simulink model "ssm"  (R2017b)
settings: Solver=FixedStepDiscrete  StartTime=0.0  StopTime=20  FixedStep=T_s_power  MaxStep=1e-4  RelTol=1e-3
values from neighbouring files (symbols this model uses):
  F_b = 50.0    (= 50)    [ssm_ini.m]
  L_1 = 10e-3    (= 0.01)    [ssm_ini.m]
  L_2 = 1e-3    (= 0.001)    [ssm_ini.m]
  Omega_b = 2*pi*50    (= 314.159265359)    [ssm_ini.m]
  params_abc = [S_b,U_b,Omega_b,K,K_d]    [ssm_ini.m]
  params_pll = [K_p,Omega_b]    [ssm_ini.m]
  params_pu = [S_b,U_b,Omega_b,R_pu,X_pu,H,D]    [ssm_ini.m]
  R_1 = 1.0    (= 1)    [ssm_ini.m]
  R_2 = 1.0    (= 1)    [ssm_ini.m]
  S_b = 20e3    (= 20000)    [ssm_ini.m]
  T_s_control = 100e-6    (= 0.0001)    [ssm_ini.m]
  T_s_power = 100e-6    (= 0.0001)    [ssm_ini.m]
undefined symbols (not defined in the file or in its folder): DiscIntNeverNeededParam
libraries: powerlib x18, powerlib_meascontrol x6
settings Model: Creator=jmmauricio  LastModifiedBy=jmmau
settings CodeAppCC: StateflowObjectComments=on
settings SimscapeCC: SimscapeNormalizeSystem=off

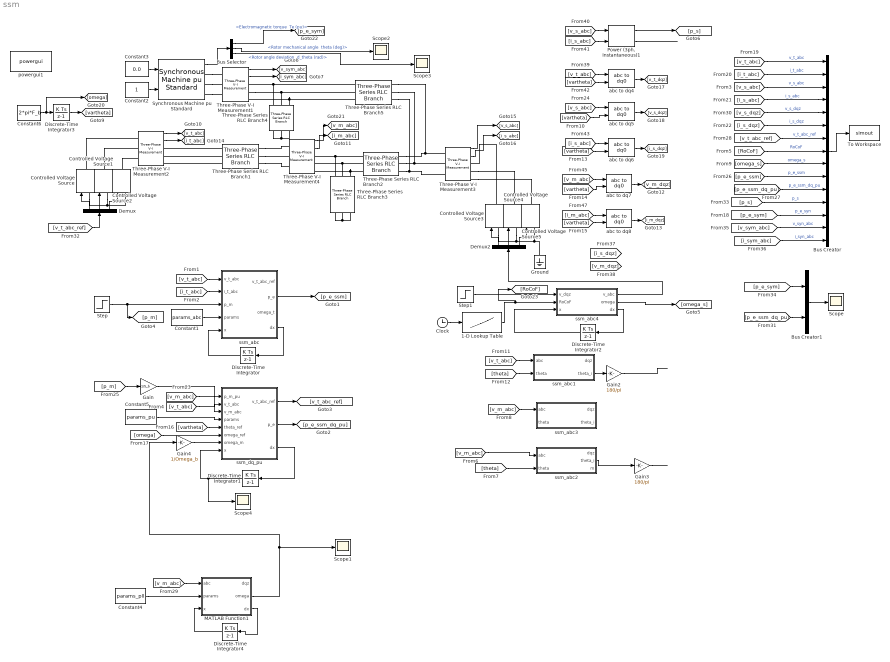
== system ssm ==
  1-D Lookup Table : Lookup_n-D  NumberOfTableDimensions=1  BreakpointsForDimension1=[0,1,1.01,6.0,6.01,15]+5  Table=[0,0,-1,-1,0,0]  InternalRulePriority=Speed  RndMeth=Simplest  InputSameDT=on
  Bus Creator : BusCreator  Inputs=15
  Bus Creator1 : BusCreator  Inputs=2
  Bus Selector : BusSelector  OutputSignals="Mechanical.Electromagnetic torque  Te (pu),Mechanical.Rotor mechanical angle  theta (deg),Mechanical.Rotor angle deviation  d_theta (rad)"
  Clock : Clock
  Constant1 : Constant  Value=params_abc
  Constant2 : Constant
  Constant3 : Constant  Value=0.0
  Constant4 : Constant  Value=params_pll
  Constant5 : Constant  Value=params_pu
  Constant6 : Constant  Value=2*pi*F_b
  Controlled Voltage Source{,1..5} (6 alike) : powerlib/Electrical Sources/Controlled Voltage Source  Initialize=on  Source_Type=AC  Amplitude=0  Phase=0  Frequency=0  Measurements=None
  Demux : Demux  Outputs=3
  Demux2 : Demux  Outputs=3
  Discrete-Time Integrator : DiscreteIntegrator  InitialCondition=[0,Omega_b]  InitialConditionSetting=State (most efficient)  SampleTime=T_s_power  ICPrevOutput=DiscIntNeverNeededParam  ICPrevScaledInput=DiscIntNeverNeededParam
  Discrete-Time Integrator1 : DiscreteIntegrator  InitialCondition=[0,1,0]  InitialConditionSetting=State (most efficient)  SampleTime=T_s_control  ICPrevOutput=DiscIntNeverNeededParam  ICPrevScaledInput=DiscIntNeverNeededParam
  Discrete-Time Integrator2 : DiscreteIntegrator  InitialCondition=[0,Omega_b]  InitialConditionSetting=State (most efficient)  SampleTime=T_s_power  ICPrevOutput=DiscIntNeverNeededParam  ICPrevScaledInput=DiscIntNeverNeededParam
  Discrete-Time Integrator3 : DiscreteIntegrator  InitialConditionSetting=State (most efficient)  SampleTime=T_s_power  ICPrevOutput=DiscIntNeverNeededParam  ICPrevScaledInput=DiscIntNeverNeededParam
  Discrete-Time Integrator4 : DiscreteIntegrator  InitialConditionSetting=State (most efficient)  SampleTime=T_s_power  ICPrevOutput=DiscIntNeverNeededParam  ICPrevScaledInput=DiscIntNeverNeededParam
  Gain : Gain  Gain=1/S_b
  Gain2 : Gain  Gain=180/pi
  Gain3 : Gain  Gain=180/pi
  Gain4 : Gain  Gain=1/Omega_b
  Ground : powerlib/Elements/Ground  LConnTagsString=a
  MATLAB Function1 : MATLAB Function  TreatAsAtomicUnit=on
  "Power (3ph, Instantaneous)1" : powerlib_meascontrol/Measurements/Power (3ph, Instantaneous)
      settings: SourceProductName=Simscape Power Systems
  Scope{,1..4} (5 alike) : Scope
  Step : Step  After=0  SampleTime=0
  Step1 : Step  Before=[0,-400*sqrt(2/3),0]  After=[0,-400*sqrt(2/3),0]  SampleTime=0
  Synchronous Machine pu Standard : powerlib/Machines/Synchronous Machine pu Standard  PresetModel=No  MechanicalLoad=Mechanical power Pm  ShowDetailedParameters=on  RotorType=Salient-pole  Units=per unit standard parameters  MeasurementBus=off  NominalParameters=[2e+04 400 50]  Reactances1=[ 1.81, 0.3, 0.23, 1.76, 0.65, 0.25, 0.15 ]  Reactances2=[1.56 0.15 0.11 0.78 0.17 0.063]  dAxisTimeConstants=Short-circuit  qAxisTimeConstants=Short-circuit  TimeConstants1="[ 5  0.1  0.1  ]"  TimeConstants2=[ 8.0, 0.03, 1.0, 0.07 ]  TimeConstants3="[  4.49  0.0681  0.0513  ]"  TimeConstants4=[ 8.0, 0.03, 0.3371, 0.0295 ]  TimeConstants5=[ 1.01, 0.053, 0.1 ]  TimeConstants6=[ 1.3201, 0.023, 1.0, 0.07 ]  TimeConstants7=[0.024 0.006 0.006]  TimeConstants8=[ 1.3201, 0.0231, 0.3371, 0.0295 ]  StatorResistance=0.0  Mechanical=[5.0 0.0 2]  PolePairs=2  InitialConditions="[ 0  -90  0  0  0  0  0  0  1 ]"  SetSaturation=off  Saturation=[0.6404,0.7127,0.8441,0.9214,0.9956,1.082,1.19,1.316,1.457;0.7,0.7698,0.8872,0.9466,0.9969,1.046,1.1,1.151,1.201]  LoadFlowParameters=[1 0 0 0 0]  TsPowergui=0  TsBlock=-1  IterativeModel=Trapezoidal non iterative  IterativeDiscreteModel=Trapezoidal non iterative  BusType=PV  Pref=30e3  Qref=0  Qmin=-inf  Qmax=inf  PLF=0  QLF=0
      settings: SourceProductName=Simscape Power Systems
  Three-Phase Series RLC Branch1 : powerlib/Elements/Three-Phase Series RLC Branch  LConnTagsString=A|B|C  RConnTagsString=A|B|C  BranchType=RL  Resistance=R_1  Inductance=L_1  Capacitance=1e-6  Measurements=None
  Three-Phase Series RLC Branch2 : powerlib/Elements/Three-Phase Series RLC Branch  LConnTagsString=A|B|C  RConnTagsString=A|B|C  BranchType=RL  Resistance=R_2  Inductance=L_2  Capacitance=1e-6  Measurements=None
  Three-Phase Series RLC Branch3 : powerlib/Elements/Three-Phase Series RLC Branch  LConnTagsString=A|B|C  RConnTagsString=A|B|C  BranchType=R  Resistance=1e2  Inductance=L_1  Capacitance=1e-6  Measurements=None
  Three-Phase Series RLC Branch4 : powerlib/Elements/Three-Phase Series RLC Branch  LConnTagsString=A|B|C  RConnTagsString=A|B|C  BranchType=R  Resistance=1e3  Inductance=L_1  Capacitance=1e-6  Measurements=None
  Three-Phase Series RLC Branch5 : powerlib/Elements/Three-Phase Series RLC Branch  LConnTagsString=A|B|C  RConnTagsString=A|B|C  BranchType=RL  Resistance=R_2  Inductance=L_2  Capacitance=1e-6  Measurements=None
  Three-Phase V-I Measurement{1..4} (4 alike) : powerlib/Measurements/Three-Phase V-I Measurement  VoltageMeasurement=phase-to-ground  SetLabelV=off  LabelV=Vabc  Vpu=off  VpuLL=off  CurrentMeasurement=yes  SetLabelI=off  LabelI=Iabc  Ipu=off  Pbase=100e6  Vbase=500e3  OutputType=Complex  PhasorSimulation=off  PSBequivalent=0
  To Workspace : ToWorkspace  VariableName=simout  SaveFormat=Timeseries  SampleTime=0.001
  abc to dq{4..8} (5 alike) : powerlib_meascontrol/Transformations/abc to dq0  Alignment=Aligned with phase A axis
  powergui1 : powerlib/powergui  Priority=1  SimulationMode=Discrete  SampleTime=T_s_power  frequency=60  Iterations=50  frequencyindice=0  Pbase=100e6  ErrMax=0.0001  UnitsV=kV  UnitsW=MW  buscounter=0  FunctionMessages=off  echomessages=off  EnableUseOfTLC=off  CurrentSourceSwitches=off  DisableSnubberDevices=off  DisableRonSwitches=off  DisableVfSwitches=off  DisplayEquations=off  SolverType=Tustin/Backward Euler (TBE)  Interpol=off  ExternalGateDelay=off  methode=off  Ts=100  x0status=steady  SPID=on  SwTol=0  HookPort=off  RestoreLinks=warning  ResistiveCurrentMeasurement=off  Frange=[0:2:500]  Ylog=off  Xlog=on  ShowGrid=off  save=off  variable=ZData  structure=0  ZoomFFT=off  StartTime=0.0  cycles=1  DisplayStyle=1  fundamental=60  FreqAxis=off  MaxFrequency=1000  frequencyindicesteady=1  RmsSteady=1  display=off
  ssm_abc : MATLAB Function  TreatAsAtomicUnit=on
  ssm_abc1 : MATLAB Function  TreatAsAtomicUnit=on
  ssm_abc2 : MATLAB Function  TreatAsAtomicUnit=on
  ssm_abc3 : MATLAB Function  TreatAsAtomicUnit=on
  ssm_abc4 : MATLAB Function  TreatAsAtomicUnit=on
  ssm_dq_pu : MATLAB Function  TreatAsAtomicUnit=on
  wires:
  Constant1/1 -> ssm_abc/4(params)
  Discrete-Time Integrator/1 -> ssm_abc/5(x)
  ssm_abc/4(dx) -> Discrete-Time Integrator/1
  Three-Phase V-I Measurement3/2 -> [i_s_abc]
  [i_s_abc] -> "Power (3ph, Instantaneous)1"/2
  abc to dq4/1 -> [v_t_dqz]
  [v_s_dqz] -> Bus Creator/5  "v_s_dqz"
  Three-Phase V-I Measurement2/1 -> [v_t_abc]
  "Power (3ph, Instantaneous)1"/2 -> ?
  Three-Phase V-I Measurement4/1 -> [v_m_abc]
  [v_s_abc] -> abc to dq5/1
  [vartheta] -> abc to dq7/2
  Demux/2 -> Controlled Voltage Source1/1
  "Power (3ph, Instantaneous)1"/1 -> [p_s]
  abc to dq6/1 -> [i_s_dqz]
  abc to dq7/1 -> [v_m_dqz]
  [v_m_abc] -> abc to dq7/1
  [vartheta] -> abc to dq8/2
  [i_s_abc] -> abc to dq6/1
  [v_t_abc] -> abc to dq4/1
  Discrete-Time Integrator3/1 -> [vartheta]
  abc to dq8/1 -> [i_m_dqz]
  Constant6/1 -> Discrete-Time Integrator3/1, [omega]
  Demux/1 -> Controlled Voltage Source/1
  [vartheta] -> abc to dq4/2
  Three-Phase V-I Measurement3/1 -> [v_s_abc]
  Three-Phase V-I Measurement4/2 -> [i_m_abc]
  Three-Phase V-I Measurement2/2 -> [i_t_abc]
  Demux/3 -> Controlled Voltage Source2/1
  abc to dq5/1 -> [v_s_dqz]
  [i_m_abc] -> abc to dq8/1
  [vartheta] -> abc to dq6/2
  [v_s_abc] -> "Power (3ph, Instantaneous)1"/1
  [vartheta] -> abc to dq5/2
  Step/1 -> [p_m], ssm_abc/3(p_m)
  [v_t_abc] -> ssm_abc/1(v_t_abc)
  [i_t_abc] -> ssm_abc/2(i_t_abc)
  ssm_abc/2(p_e) -> [p_e_ssm]
  Constant5/1 -> ssm_dq_pu/4(params)
  [v_m_abc] -> ssm_dq_pu/3(v_m_abc)
  [v_t_abc] -> ssm_dq_pu/2(v_t_abc)
  Gain/1 -> ssm_dq_pu/1(p_m_pu)
  Discrete-Time Integrator1/1 -> Scope4/1, ssm_dq_pu/8(x)
  ssm_dq_pu/3(dx) -> Discrete-Time Integrator1/1
  [v_t_abc] -> ssm_abc1/1(abc)
  [theta] -> ssm_abc1/2(theta)
  ssm_abc1/2(theta_i) -> Gain2/1
  Gain2/1 -> ?
  [v_m_abc] -> ssm_abc2/1(abc)
  [theta] -> ssm_abc2/2(theta)
  Gain3/1 -> ?
  ssm_abc2/2(theta_i) -> Gain3/1
  [v_m_abc] -> ssm_abc3/1(abc)
  [vartheta] -> ssm_dq_pu/5(theta_ref)
  [omega] -> ssm_dq_pu/6(omega_ref)
  Demux2/3 -> Controlled Voltage Source5/1
  Demux2/2 -> Controlled Voltage Source4/1
  Demux2/1 -> Controlled Voltage Source3/1
  ssm_abc4/1(v_abc) -> Demux2/1
  Discrete-Time Integrator2/1 -> ssm_abc4/3(x)
  ssm_abc4/3(dx) -> Discrete-Time Integrator2/1
  Step1/1 -> ssm_abc4/1(v_dqz)
  MATLAB Function1/2(omega) -> Scope1/1, Gain4/1
  Gain4/1 -> ssm_dq_pu/7(omega_m)
  1-D Lookup Table/1 -> [RoCoF], ssm_abc4/2(RoCoF)
  Bus Creator/1 -> To Workspace/1
  [v_t_abc] -> Bus Creator/1  "v_t_abc"
  [i_t_abc] -> Bus Creator/2  "i_t_abc"
  [v_s_abc] -> Bus Creator/3  "v_s_abc"
  [i_s_abc] -> Bus Creator/4  "i_s_abc"
  [i_s_dqz] -> Bus Creator/6  "i_s_dqz"
  ssm_dq_pu/2(p_e) -> [p_e_ssm_dq_pu]
  ssm_dq_pu/1(v_t_abc_ref) -> [v_t_abc_ref]
  [p_m] -> Gain/1
  Clock/1 -> 1-D Lookup Table/1
  ssm_abc4/2(omega) -> [omega_s]
  [RoCoF] -> Bus Creator/8  "RoCoF"
  [omega_s] -> Bus Creator/9  "omega_s"
  [p_e_ssm] -> Bus Creator/10  "p_e_ssm"
  [p_e_ssm_dq_pu] -> Bus Creator/11  "p_e_ssm_dq_pu"
  [v_t_abc_ref] -> Bus Creator/7  "v_t_abc_ref"
  [p_s] -> Bus Creator/12  "p_s"
  [v_t_abc_ref] -> Demux/1
  Three-Phase V-I Measurement1/1 -> [v_sym_abc]
  Three-Phase V-I Measurement1/2 -> [i_sym_abc]
  Synchronous Machine pu Standard/1 -> Bus Selector/1
  Bus Selector/1 -> [p_e_sym]  "<Electromagnetic torque  Te (pu)>"
  Bus Creator1/1 -> Scope/1
  [p_e_ssm_dq_pu] -> Bus Creator1/2
  [p_e_sym] -> Bus Creator1/1
  Constant2/1 -> Synchronous Machine pu Standard/2
  Constant3/1 -> Synchronous Machine pu Standard/1
  Discrete-Time Integrator4/1 -> MATLAB Function1/3(x)
  Constant4/1 -> MATLAB Function1/2(params)
  MATLAB Function1/3(dx) -> Discrete-Time Integrator4/1
  [v_m_abc] -> MATLAB Function1/1(abc)
  Bus Selector/2 -> Scope2/1  "<Rotor mechanical angle  theta (deg)>"
  Bus Selector/3 -> Scope3/1  "<Rotor angle deviation  d_theta (rad)>"
  [p_e_sym] -> Bus Creator/13  "p_e_syn"
  [v_sym_abc] -> Bus Creator/14  "v_syn_abc"
  [i_sym_abc] -> Bus Creator/15  "i_syn_abc"
  connections:
  Controlled Voltage Source2/LConn1 -- Controlled Voltage Source/LConn1 -- Controlled Voltage Source1/LConn1
  Controlled Voltage Source2/RConn1 -- Three-Phase V-I Measurement2/LConn3
  Three-Phase V-I Measurement3/RConn2 -- Controlled Voltage Source4/RConn1
  Three-Phase Series RLC Branch2/LConn2 -- Three-Phase Series RLC Branch3/LConn2 -- Three-Phase V-I Measurement4/RConn2
  Three-Phase Series RLC Branch2/LConn3 -- Three-Phase Series RLC Branch3/LConn3 -- Three-Phase V-I Measurement4/RConn3
  Three-Phase Series RLC Branch2/RConn1 -- Three-Phase Series RLC Branch5/RConn1 -- Three-Phase V-I Measurement3/LConn1
  Controlled Voltage Source/RConn1 -- Three-Phase V-I Measurement2/LConn1
  Three-Phase Series RLC Branch2/RConn2 -- Three-Phase Series RLC Branch5/RConn2 -- Three-Phase V-I Measurement3/LConn2
  Controlled Voltage Source3/RConn1 -- Three-Phase V-I Measurement3/RConn1
  Three-Phase Series RLC Branch1/LConn2 -- Three-Phase V-I Measurement2/RConn2
  Three-Phase Series RLC Branch2/LConn1 -- Three-Phase Series RLC Branch3/LConn1 -- Three-Phase V-I Measurement4/RConn1
  Controlled Voltage Source1/RConn1 -- Three-Phase V-I Measurement2/LConn2
  Three-Phase Series RLC Branch1/LConn3 -- Three-Phase V-I Measurement2/RConn3
  Three-Phase Series RLC Branch1/RConn2 -- Three-Phase V-I Measurement4/LConn2
  Three-Phase V-I Measurement3/RConn3 -- Controlled Voltage Source5/RConn1
  Three-Phase Series RLC Branch1/LConn1 -- Three-Phase V-I Measurement2/RConn1
  Three-Phase Series RLC Branch1/RConn3 -- Three-Phase V-I Measurement4/LConn3
  Three-Phase Series RLC Branch2/RConn3 -- Three-Phase Series RLC Branch5/RConn3 -- Three-Phase V-I Measurement3/LConn3
  Three-Phase Series RLC Branch1/RConn1 -- Three-Phase V-I Measurement4/LConn1
  Controlled Voltage Source4/LConn1 -- Ground/LConn1 -- Controlled Voltage Source5/LConn1 -- Controlled Voltage Source3/LConn1
  Synchronous Machine pu Standard/RConn1 -- Three-Phase V-I Measurement1/LConn1
  Synchronous Machine pu Standard/RConn2 -- Three-Phase V-I Measurement1/LConn2
  Synchronous Machine pu Standard/RConn3 -- Three-Phase V-I Measurement1/LConn3
  Three-Phase Series RLC Branch3/RConn1 -- Three-Phase Series RLC Branch3/RConn2 -- Three-Phase Series RLC Branch3/RConn3
  Three-Phase Series RLC Branch5/LConn1 -- Three-Phase Series RLC Branch4/LConn1 -- Three-Phase V-I Measurement1/RConn1
  Three-Phase V-I Measurement1/RConn2 -- Three-Phase Series RLC Branch4/LConn2 -- Three-Phase Series RLC Branch5/LConn2
  Three-Phase Series RLC Branch5/LConn3 -- Three-Phase Series RLC Branch4/LConn3 -- Three-Phase V-I Measurement1/RConn3
  Three-Phase Series RLC Branch4/RConn1 -- Three-Phase Series RLC Branch4/RConn2 -- Three-Phase Series RLC Branch4/RConn3

== matlab function ssm/ssm_abc1 ==
  data: abc input; dqz output; theta_i output; theta input
function [dqz,theta_i] = fcn(abc,theta)


T_p = 2.0/3.0*[[ cos(theta), cos(theta-2.0/3.0*pi), cos(theta+2.0/3.0*pi)],
               [-sin(theta),-sin(theta-2.0/3.0*pi),-sin(theta+2.0/3.0*pi)],
               [        0.5,                   0.5,                   0.5]];
           
dqz = T_p *abc;

theta_i = atan2(dqz(1),-dqz(2));

== matlab function ssm/ssm_abc ==
  data: v_t_abc input; i_t_abc input; p_m input; params input; v_t_abc_ref output; p_e output; omega_t output; x input; dx output
function [v_t_abc_ref,p_e,omega_t,dx] = fcn(v_t_abc,i_t_abc,p_m,params,x)

Omega_b = 2*pi*50;
V_t = 400.0*sqrt(2/3);
p_e = sum(v_t_abc.*i_t_abc);


theta_t = x(1);
omega_t = x(2);

K   = params(4);
K_d = params(5);

dtheta_t = omega_t;
domega_t = K*(p_m - p_e -(omega_t-Omega_b)*K_d);

v_t_abc_ref = V_t * [sin(theta_t), sin(theta_t-2.0/3.0*pi), sin(theta_t-4.0/3.0*pi)].';

dx = [dtheta_t; domega_t];

== matlab function ssm/ssm_abc2 ==
  data: abc input; dqz output; theta_i output; theta input; m output
function [dqz,theta_i,m] = fcn(abc,theta)


T_p = 2.0/3.0*[[ cos(theta), cos(theta-2.0/3.0*pi), cos(theta+2.0/3.0*pi)],
               [-sin(theta),-sin(theta-2.0/3.0*pi),-sin(theta+2.0/3.0*pi)],
               [        0.5,                   0.5,                   0.5]];
           
dqz = T_p *abc;

theta_i = atan2(dqz(1),-dqz(2));
m = sqrt(dqz(1)^2+dqz(2)^2);

== matlab function ssm/ssm_dq_pu ==
  data: p_m_pu input; v_t_abc input; v_t_abc_ref output; p_e output; v_m_abc input; params input; theta_ref input; omega_ref input; omega_m input; dx output; x input
function [v_t_abc_ref,p_e,dx] = fcn(p_m_pu,v_t_abc,v_m_abc,params,theta_ref,omega_ref,omega_m,x)

S_b = params(1);
U_b = params(2);
Omega_b = params(3);
R_pu = params(4);
X_pu = params(5);
H = params(6);
D = params(7);

v_t_dqz_ref = [0.0, 0.0, 0].';

V_b_dq = U_b*sqrt(2/3);
I_b_dq = S_b/U_b*sqrt(2/3);


delta = x(1);
omega_t = x(2);
omega_mp = x(3);

theta = theta_ref;

T_p = 2.0/3.0*[[ cos(theta), cos(theta-2.0/3.0*pi), cos(theta+2.0/3.0*pi)],
               [-sin(theta),-sin(theta-2.0/3.0*pi),-sin(theta+2.0/3.0*pi)],
               [        0.5,                   0.5,                   0.5]];
           

T_p_inv = [[            cos(theta),            -sin(theta), 1.0],
           [ cos(theta-2.0/3.0*pi), -sin(theta-2.0/3.0*pi), 1.0],
           [ cos(theta+2.0/3.0*pi), -sin(theta+2.0/3.0*pi), 1.0]];

v_t_dqz = T_p * v_t_abc;
v_m_dqz = T_p * v_m_abc;

v_t_d_pu =  v_t_dqz(1)/V_b_dq; % slack (Kron's) reference frame 
v_t_q_pu =  v_t_dqz(2)/V_b_dq; % slack (Kron's) reference frame 

v_m_d_pu =  v_m_dqz(1)/V_b_dq; % slack (Kron's) reference frame
v_m_q_pu =  v_m_dqz(2)/V_b_dq; % slack (Kron's) reference frame

theta = delta;

v_td = cos(theta)*v_t_d_pu + cos(theta-pi/2)*v_t_q_pu;
v_tq =-sin(theta)*v_t_d_pu - sin(theta-pi/2)*v_t_q_pu;
v_md = cos(theta)*v_m_d_pu + cos(theta-pi/2)*v_m_q_pu;
v_mq =-sin(theta)*v_m_d_pu - sin(theta-pi/2)*v_m_q_pu;


i_d = -(R_pu*(v_md - v_td) + X_pu*(v_mq -v_tq))/(X_pu^2 + R_pu^2); % slack (Kron's) reference frame
i_q = -(R_pu*(v_mq - v_tq) - X_pu*(v_md -v_td))/(X_pu^2 + R_pu^2); % slack (Kron's) reference frame

p_e = v_td*i_d + v_tq*i_q;

ddelta = Omega_b*(omega_t-1);
domega_t = 1/(2*H)*(p_m_pu - p_e -(omega_t-omega_m)*D);
domega_mp = 1*((omega_t-1)-omega_mp);
v_td_ref =  0.0;
v_tq_ref = -1.0;

theta = -delta;
v_td_ref_k = cos(theta)*v_td_ref + cos(theta-pi/2)*v_tq_ref; % Kron reference frame
v_tq_ref_k =-sin(theta)*v_td_ref - sin(theta-pi/2)*v_tq_ref; % Kron reference frame

v_t_dqz_ref_k = [v_td_ref_k, v_tq_ref_k, 0].';

v_t_abc_ref = T_p_inv * v_t_dqz_ref_k * V_b_dq;  % abc 

dx = [ddelta; domega_t;domega_mp];

== matlab function ssm/ssm_abc3 ==
  data: abc input; dqz output; theta_i output; theta input
function [dqz,theta_i] = fcn(abc,theta)


T_p = 2.0/3.0*[[ cos(theta), cos(theta-2.0/3.0*pi), cos(theta+2.0/3.0*pi)],
               [-sin(theta),-sin(theta-2.0/3.0*pi),-sin(theta+2.0/3.0*pi)],
               [        0.5,                   0.5,                   0.5]];
           
dqz = T_p *abc;

theta_i = atan2(dqz(1),-dqz(2));

== matlab function ssm/ssm_abc4 ==
  data: v_dqz input; v_abc output; omega output; RoCoF input; dx output; x input
function [v_abc,omega,dx] = fcn(v_dqz,RoCoF,x)

theta = x(1);
omega = x(2);

T_p_inv = [[            cos(theta),            -sin(theta), 1.0],
           [ cos(theta-2.0/3.0*pi), -sin(theta-2.0/3.0*pi), 1.0],
           [ cos(theta+2.0/3.0*pi), -sin(theta+2.0/3.0*pi), 1.0]];


dtheta = omega;
domega = 2*pi*RoCoF; % RoCoF in Hz/s, omega in rad/s

v_abc = T_p_inv*v_dqz;

dx = [dtheta,domega];

== matlab function ssm/MATLAB Function1 ==
  data: abc input; dqz output; omega output; params input; x input; dx output
function [dqz,omega,dx] = pll(abc,params,x)

K_p = params(1);
Omega_b = params(2);



theta = x(1);
T_p = 2.0/3.0*[[ cos(theta), cos(theta-2.0/3.0*pi), cos(theta+2.0/3.0*pi)],
               [-sin(theta),-sin(theta-2.0/3.0*pi),-sin(theta+2.0/3.0*pi)],
               [        0.5,                   0.5,                   0.5]];

dqz = T_p * abc;
           


omega = K_p*dqz(2) + Omega_b;

dtheta = omega;

dx = [dtheta];
